simulink model "simulink1"  (R2013a)
settings: Solver=ode45  StartTime=0.0  StopTime=10.0  RelTol=1e-3  AbsTol=1e-6
values from neighbouring files (symbols this model uses):
  a0 = Wn*2    (= 6)    [Skoki.m]    (also in symulek1.m = 1)
  a1 = Aw1*sqrt(2*g*h1max)/h1max    [Kaskady.m]    (also in Kaskady2.m; Skoki.m = 2*Wn*ksi(i); symulek1.m = 1; transmitacje.m)
  b = 1    [Skoki.m]    (also in symulek1.m = 9)
  du = 1    [Skoki.m]    (also in symulek1.m)
  t0 = 1    [Kaskady.m]    (also in Kaskady2.m; Skoki.m = 0; symulek1.m; transmitacje.m)
  u0 = 0    [Skoki.m]    (also in symulek1.m)
  x0 = 0    [Skoki.m]    (also in symulek1.m)
settings Model: Creator=LAB320-1552  LastModifiedBy=pc
settings DebuggingCC: SolverPrmCheckMsg=none

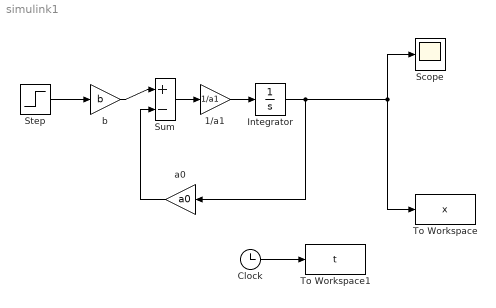
== system simulink1 ==
  1/a1 : Gain  Gain=1/a1
  Clock : Clock
  Integrator : Integrator  InitialCondition=x0
  Scope : Scope
  Step : Step  Time=t0  Before=u0  After=u0+du  SampleTime=0
  Sum : Sum  Inputs=|+-
  To Workspace : ToWorkspace  VariableName=x  SampleTime=-1
  To Workspace1 : ToWorkspace  VariableName=t  SampleTime=-1
  a0 : Gain  Gain=a0
  "b " : Gain  Gain=b
  wires:
  Step/1 -> "b "/1
  Sum/1 -> 1/a1/1
  1/a1/1 -> Integrator/1
  Integrator/1 -> To Workspace/1, Scope/1, a0/1
  a0/1 -> Sum/2
  "b "/1 -> Sum/1
  Clock/1 -> To Workspace1/1
